simulink model "4_bit_Binary_Password_Finder_using_JK_Flip_Flop_and_Sequential_Logic"  (R2022b)
settings: Solver=VariableStepAuto  StartTime=0.0  StopTime=32  RelTol=1e-3
libraries: simulink_extras x5
settings Model: Creator=Hüseyin Keskin  LastModifiedBy=Hüseyin Keskin

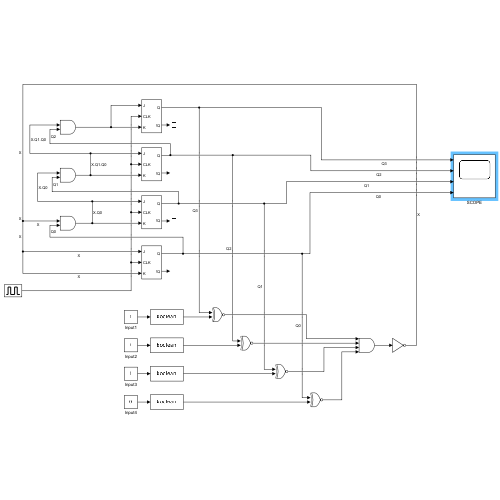
[thumbnail: Simulink's stored preview of the top-level diagram]
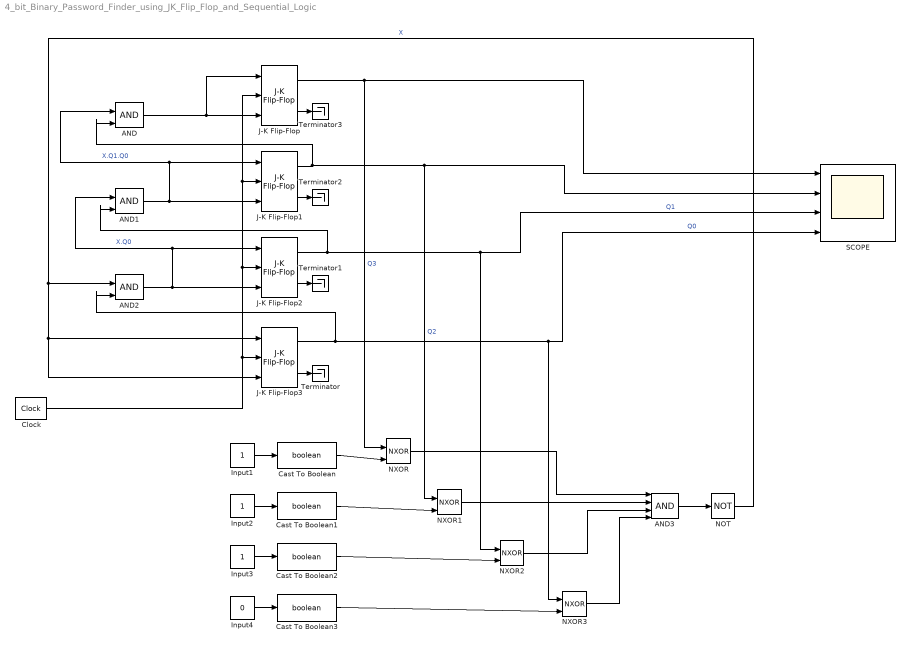
== system 4_bit_Binary_Password_Finder_using_JK_Flip_Flop_and_Sequential_Logic ==
  AND : Logic  IconShape=distinctive  AllPortsSameDT=off  OutDataTypeStr=boolean
  AND1 : Logic  IconShape=distinctive  AllPortsSameDT=off  OutDataTypeStr=boolean
  AND2 : Logic  IconShape=distinctive  AllPortsSameDT=off  OutDataTypeStr=boolean
  AND3 : Logic  Inputs=4  IconShape=distinctive  AllPortsSameDT=off  OutDataTypeStr=boolean
  Cast To Boolean{,1..3} (4 alike) : DataTypeConversion  OutDataTypeStr=boolean  SaturateOnIntegerOverflow=off  RndMeth=Floor
  Clock : simulink_extras/Flip Flops/Clock  period=2
  Input1 : Constant
  Input2 : Constant
  Input3 : Constant
  Input4 : Constant  Value=0
  J-K Flip-Flop{,1..3} (4 alike) : simulink_extras/Flip Flops/J-K Flip-Flop  initial_condition=0
  NOT : Logic  Operator=NOT  IconShape=distinctive  AllPortsSameDT=off  OutDataTypeStr=boolean
  NXOR{,1..3} (4 alike) : Logic  Operator=NXOR  IconShape=distinctive  AllPortsSameDT=off  OutDataTypeStr=boolean
  SCOPE : Scope  NumInputPorts=4
  Terminator{,1..3} (4 alike) : Terminator
  wires:
  J-K Flip-Flop3/2 -> Terminator/1
  J-K Flip-Flop2/2 -> Terminator1/1
  J-K Flip-Flop1/2 -> Terminator2/1
  J-K Flip-Flop/2 -> Terminator3/1
  AND/1 -> J-K Flip-Flop/3, J-K Flip-Flop/1
  Clock/1 -> J-K Flip-Flop3/2, J-K Flip-Flop2/2, J-K Flip-Flop1/2, J-K Flip-Flop/2
  J-K Flip-Flop/1 -> SCOPE/1, NXOR/1  "Q3"
  J-K Flip-Flop3/1 -> SCOPE/4, NXOR3/1, AND2/2  "Q0"
  NOT/1 -> AND2/1, J-K Flip-Flop3/1, J-K Flip-Flop3/3  "X"
  AND3/1 -> NOT/1
  NXOR/1 -> AND3/1
  NXOR1/1 -> AND3/2
  NXOR2/1 -> AND3/3
  NXOR3/1 -> AND3/4
  Input1/1 -> Cast To Boolean/1
  Input2/1 -> Cast To Boolean1/1
  Input3/1 -> Cast To Boolean2/1
  Input4/1 -> Cast To Boolean3/1
  J-K Flip-Flop1/1 -> AND/2, NXOR1/1, SCOPE/2  "Q2"
  J-K Flip-Flop2/1 -> SCOPE/3, NXOR2/1, AND1/2  "Q1"
  AND2/1 -> J-K Flip-Flop2/3, J-K Flip-Flop2/1, AND1/1  "X.Q0"
  AND1/1 -> J-K Flip-Flop1/1, AND/1, J-K Flip-Flop1/3  "X.Q1.Q0"
  Cast To Boolean/1 -> NXOR/2
  Cast To Boolean3/1 -> NXOR3/2
  Cast To Boolean2/1 -> NXOR2/2
  Cast To Boolean1/1 -> NXOR1/2
